simulink model "model_HO"  (R2023b)
settings: Solver=FixedStepAuto  StartTime=0.0  StopTime=119.99  FixedStep=0.01  RelTol=1e-3
values from neighbouring files (symbols this model uses):
  b = 0.22    [init_model_HO.m]
  fofu_nr = 1    [init_model_HO.m]
  fofu_tab = table2array(fofu_tab)    [init_model_HO.m]
  H_ce = tf([0 K_ce], [1 0 0])    [init_model_HO.m]
  H_star = (H_oe*H_nms*inv_stick)    [init_model_HO.m]
  I = 0.01    [init_model_HO.m]
  k = 3.58    [init_model_HO.m]
  K_f = 1.07    [init_model_HO.m]
  K_HO = K_HO_    [init_model_HO.m]
  K_n = 0    [init_model_HO.m]
  K_stick = 10    [init_model_HO.m]
  T_lf = 0.95    [init_model_HO.m]
  tau_p = tau_p_    [init_model_HO.m]
  tau_v = 0.33    [init_model_HO.m]
  w_bn = 1/0.23    (= 4.34782608696)    [init_model_HO.m]
libraries: simulink x1
settings Model: Creator=cgome  LastModifiedBy=mihai

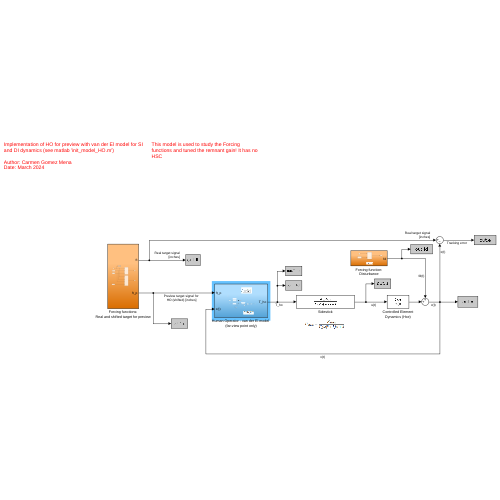
[thumbnail: Simulink's stored preview of the top-level diagram]
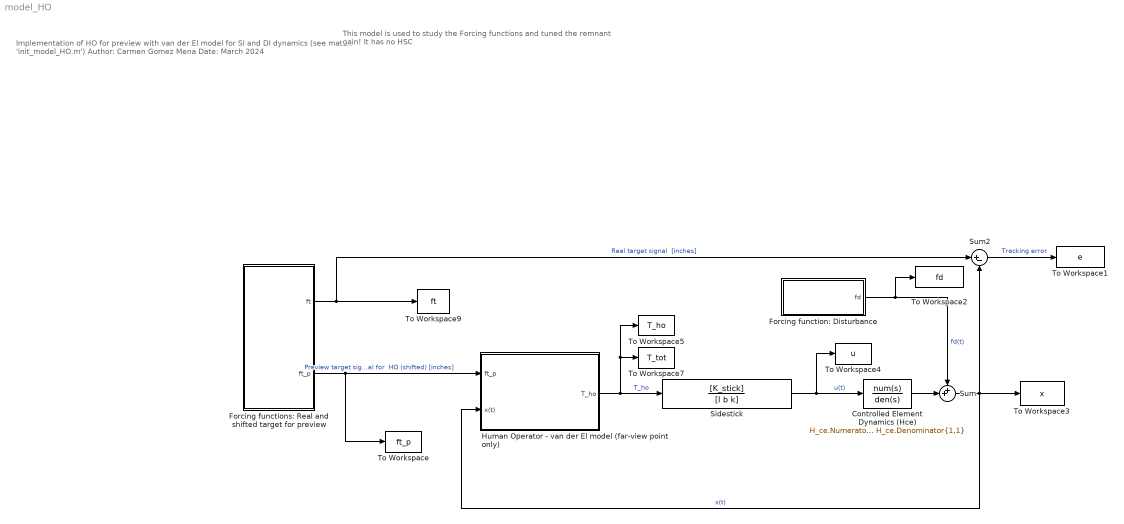
== system model_HO ==
  note: Implementation of HO for preview with van der El model for SI and DI dynamics (see matlab 'init_model_HO.m')
      |
      | Author: Carmen Gomez Mena
      | Date: March 2024
  note: This model is used to study the Forcing functions and tuned the remnant gain! It has no HSC
  Controlled Element Dynamics (Hce) : TransferFcn  Numerator=H_ce.Numerator{1,1}  Denominator=H_ce.Denominator{1,1}
  Forcing function: Disturbance : Subsystem
  Forcing functions: Real and shifted target for preview : Subsystem
  Human Operator - van der El model (far-view point only) : Subsystem
  Sidestick : TransferFcn  Numerator=[K_stick]  Denominator=[I b k]
  Sum : Sum  Inputs=++|
  Sum2 : Sum  Inputs=|+-
  To Workspace : ToWorkspace  VariableName=ft_p  SaveFormat=Timeseries  SampleTime=-1
  To Workspace1 : ToWorkspace  VariableName=e  SaveFormat=Timeseries  SampleTime=-1
  To Workspace2 : ToWorkspace  VariableName=fd  SaveFormat=Timeseries  SampleTime=-1
  To Workspace3 : ToWorkspace  VariableName=x  SaveFormat=Timeseries  SampleTime=-1
  To Workspace4 : ToWorkspace  VariableName=u  SaveFormat=Timeseries  SampleTime=-1
  To Workspace5 : ToWorkspace  VariableName=T_ho  SaveFormat=Timeseries  SampleTime=-1
  To Workspace7 : ToWorkspace  VariableName=T_tot  SaveFormat=Timeseries  SampleTime=-1
  To Workspace9 : ToWorkspace  VariableName=ft  SaveFormat=Timeseries  SampleTime=-1
  wires:
  Forcing functions: Real and shifted target for preview/2(ft_p) -> Human Operator - van der El model (far-view point only)/1(ft_p), To Workspace/1  "Preview target signal for  HO (shifted) [inches]"
  Forcing function: Disturbance/1(fd) -> Sum/1, To Workspace2/1  "fd(t)"
  Human Operator - van der El model (far-view point only)/1(T_ho) -> To Workspace7/1, To Workspace5/1, Sidestick/1  "T_ho"
  Sidestick/1 -> Controlled Element Dynamics (Hce)/1, To Workspace4/1  "u(t)"
  Controlled Element Dynamics (Hce)/1 -> Sum/2
  Sum2/1 -> To Workspace1/1  "Tracking error"
  Forcing functions: Real and shifted target for preview/1(ft) -> To Workspace9/1, Sum2/1  "Real target signal  [inches]"
  Sum/1 -> Human Operator - van der El model (far-view point only)/2(x(t)), To Workspace3/1, Sum2/2  "x(t)"

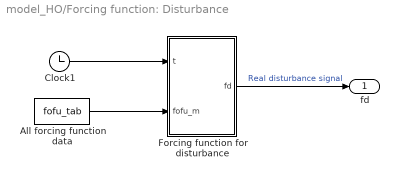
== system model_HO/Forcing function: Disturbance ==
  All forcing function data : Constant  Value=fofu_tab  VectorParams1D=off
  Clock1 : Clock
  Forcing function for disturbance : MATLAB Function  TreatAsAtomicUnit=on
  fd : Outport
  wires:
  Forcing function for disturbance/1(fd) -> fd/1  "Real disturbance signal"
  Clock1/1 -> Forcing function for disturbance/1(t)
  All forcing function data/1 -> Forcing function for disturbance/2(fofu_m)

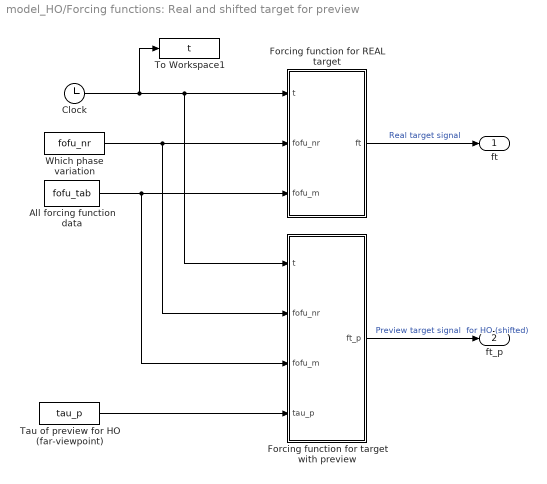
== system model_HO/Forcing functions: Real and shifted target for preview ==
  All forcing function data : Constant  Value=fofu_tab  VectorParams1D=off
  Clock : Clock
  Forcing function for REAL target : MATLAB Function  TreatAsAtomicUnit=on
  Forcing function for target with preview : MATLAB Function  TreatAsAtomicUnit=on
  "Tau of preview for HO (far-viewpoint) " : Constant  Value=tau_p
  To Workspace1 : ToWorkspace  VariableName=t  SaveFormat=Timeseries  SampleTime=-1
  Which phase variation : Constant  Value=fofu_nr
  ft : Outport
  ft_p : Outport  Port=2
  wires:
  All forcing function data/1 -> Forcing function for REAL target/3(fofu_m), Forcing function for target with preview/3(fofu_m)
  Which phase variation/1 -> Forcing function for target with preview/2(fofu_nr), Forcing function for REAL target/2(fofu_nr)
  "Tau of preview for HO (far-viewpoint) "/1 -> Forcing function for target with preview/4(tau_p)
  Clock/1 -> Forcing function for target with preview/1(t), Forcing function for REAL target/1(t), To Workspace1/1
  Forcing function for target with preview/1(ft_p) -> ft_p/1  "Preview target signal  for HO (shifted)"
  Forcing function for REAL target/1(ft) -> ft/1  "Real target signal"

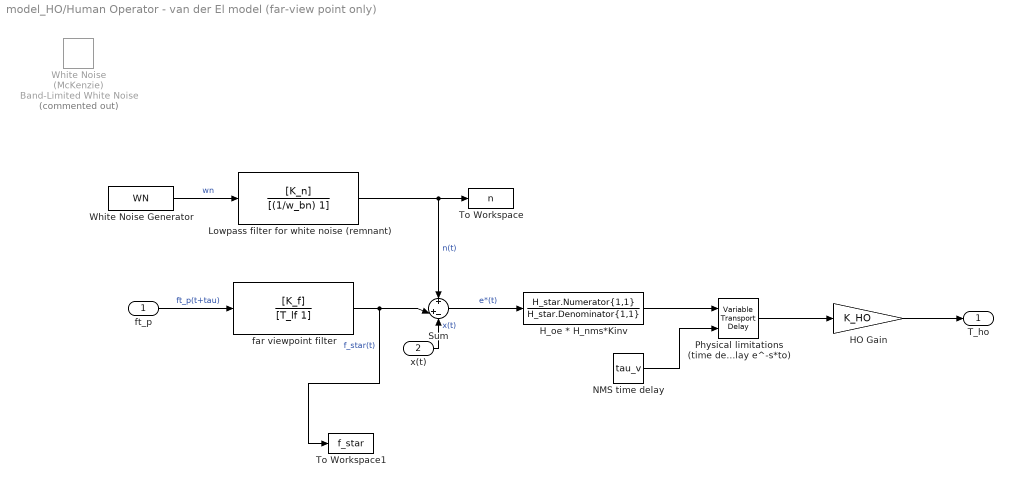
== system model_HO/Human Operator - van der El model (far-view point only) ==
  ft_p : Inport
  x(t) : Inport  Port=2
  HO Gain : Gain  Gain=K_HO
  "H_oe * H_nms*Kinv " : TransferFcn  Numerator=H_star.Numerator{1,1}  Denominator=H_star.Denominator{1,1}
  Lowpass filter for white noise (remnant) : TransferFcn  Numerator=[K_n]  Denominator=[(1/w_bn) 1]
  NMS time delay : Constant  Value=tau_v
  Physical limitations (time delay e^-s*to) : VariableTransportDelay  MaximumDelay=100
  Sum : Sum  Inputs=+|+-
  To Workspace : ToWorkspace  VariableName=n  SaveFormat=Timeseries  SampleTime=-1
  To Workspace1 : ToWorkspace  VariableName=f_star  SaveFormat=Timeseries  SampleTime=-1
  White Noise (McKenzie) : simulink/Sources/Band-Limited White Noise  Commented=on  Cov=1  Ts=0.01  seed=43786
  White Noise Generator : FromWorkspace  VariableName=WN  SampleTime=-1
  far viewpoint filter : TransferFcn  Numerator=[K_f]  Denominator=[T_lf 1]
  T_ho : Outport
  wires:
  ft_p/1 -> far viewpoint filter/1  "ft_p(t+tau)"
  Sum/1 -> "H_oe * H_nms*Kinv "/1  "e*(t)"
  "H_oe * H_nms*Kinv "/1 -> Physical limitations (time delay e^-s*to)/1
  NMS time delay/1 -> Physical limitations (time delay e^-s*to)/2
  Lowpass filter for white noise (remnant)/1 -> To Workspace/1, Sum/1  "n(t)"
  Physical limitations (time delay e^-s*to)/1 -> HO Gain/1
  x(t)/1 -> Sum/3  "x(t)"
  HO Gain/1 -> T_ho/1
  White Noise Generator/1 -> Lowpass filter for white noise (remnant)/1  "wn"
  far viewpoint filter/1 -> Sum/2, To Workspace1/1  "f_star(t)"

== matlab function model_HO/Forcing function: Disturbance/Forcing function for disturbance ==
  data: t input; fofu_m input; fd output
function fd = fcn(t, fofu_m)

fd = 0;  %initialise at 0
base_freq = 2*pi/120; 

for i=1:10 %for each of the 10 sinusoidals in the fofu data
    Ad = fofu_m(i,9); %amplitude
    % omega_d = fofu_m(i,10); %frequency
    omega_d = base_freq*fofu_m(i,8); %frequency = k*base
    phi_d = fofu_m(i,11); %phase
    
    %compute sinusoidal (no time shift)
    fd_i = Ad * sin(omega_d * (t) + phi_d);

    %Add sinuoidal to disturbance signal definition
    fd = fd + fd_i;
end

== matlab function model_HO/Forcing functions: Real and shifted target for preview/Forcing function for REAL target ==
  data: t input; ft output; fofu_nr input; fofu_m input
function ft  = fcn(t, fofu_nr, fofu_m)

ft = 0; %initialise at 0
base_freq = 2*pi/120; 

for i=1:10 %for each of the 10 sinusoidals in the fofu data
    
    At = fofu_m(i,3); %amplitude
    % omega_t = fofu_m(i,4); % frequency
    omega_t = base_freq*fofu_m(i,2); % frequency = k*base
    phi_t = fofu_m(i,4+fofu_nr); %phase (depends on fofu_nr which variation)

    %compute sinusoidal (with time shift due to preview)
    ft_i_tau = At * sin(omega_t * (t) + phi_t);
    
    %Add sinuoidal to target signal definition
    ft = ft + ft_i_tau;
end

== matlab function model_HO/Forcing functions: Real and shifted target for preview/Forcing function for target with preview ==
  data: t input; ft_p output; fofu_nr input; fofu_m input; tau_p input
function ft_p  = fcn(t, fofu_nr, fofu_m, tau_p)

ft_p = 0; %initialise at 0
base_freq = 2*pi/120; 

for i=1:10 %for each of the 10 sinusoidals in the fofu data
    
    At = fofu_m(i,3); %amplitude
    % omega_t = fofu_m(i,4); % frequency
    omega_t = base_freq*fofu_m(i,2); % frequency = k*base
    phi_t = fofu_m(i,4+fofu_nr); %phase (depends on fofu_nr which variation)

    %compute sinusoidal (with time shift due to preview)
    ft_i_tau = At * sin(omega_t * (t+tau_p) + phi_t);
    
    %Add sinuoidal to target signal definition
    ft_p = ft_p + ft_i_tau;
end
